simulink model "SIFT"  (R2013a)
settings: Solver=FixedStepDiscrete  SolverMode=SingleTasking  StartTime=0.0  StopTime=10.0  RelTol=1e-3
libraries: xbsIndex_r4 x365, xrbsImage_r4 x64
(part 10 of 10)

== system SIFT/Minima1/Subsystem ==
  In1 : Inport
  In2 : Inport  Port=2
  In4 : Inport  Port=3
  In6 : Inport  Port=4
  In8 : Inport  Port=5
  In10 : Inport  Port=6
  In12 : Inport  Port=7
  In14 : Inport  Port=8
  In16 : Inport  Port=9
  Relational{,1..7} (8 alike) : xbsIndex_r4/Relational  mode=a<b  en=off  latency=1  dbl_ovrd=off  block_type=relational
  Out1 : Outport
  Out2 : Outport  Port=2
  Out3 : Outport  Port=3
  Out4 : Outport  Port=4
  Out5 : Outport  Port=5
  Out6 : Outport  Port=6
  Out7 : Outport  Port=7
  Out8 : Outport  Port=8
  wires:
  In1/1 -> Relational7/1, Relational6/1, Relational5/1, Relational4/1, Relational3/1, Relational2/1, Relational1/1, Relational/1
  Relational/1 -> Out1/1
  In2/1 -> Relational/2
  In4/1 -> Relational1/2
  In6/1 -> Relational2/2
  In8/1 -> Relational3/2
  In10/1 -> Relational4/2
  In12/1 -> Relational5/2
  In14/1 -> Relational6/2
  In16/1 -> Relational7/2
  Relational2/1 -> Out3/1
  Relational1/1 -> Out2/1
  Relational3/1 -> Out4/1
  Relational4/1 -> Out5/1
  Relational6/1 -> Out7/1
  Relational5/1 -> Out6/1
  Relational7/1 -> Out8/1

== system SIFT/Minima1/Subsystem1 ==
  In1 : Inport
  In2 : Inport  Port=2
  In4 : Inport  Port=3
  In6 : Inport  Port=4
  In8 : Inport  Port=5
  In10 : Inport  Port=6
  In12 : Inport  Port=7
  In14 : Inport  Port=8
  In16 : Inport  Port=9
  Relational{,1..7} (8 alike) : xbsIndex_r4/Relational  mode=a<b  en=off  latency=1  dbl_ovrd=off  block_type=relational
  Out1 : Outport
  Out2 : Outport  Port=2
  Out3 : Outport  Port=3
  Out4 : Outport  Port=4
  Out5 : Outport  Port=5
  Out6 : Outport  Port=6
  Out7 : Outport  Port=7
  Out8 : Outport  Port=8
  wires:
  In1/1 -> Relational1/1, Relational7/1, Relational6/1, Relational5/1, Relational4/1, Relational3/1, Relational2/1, Relational/1
  Relational/1 -> Out1/1
  In2/1 -> Relational/2
  In4/1 -> Relational1/2
  In6/1 -> Relational7/2
  In8/1 -> Relational6/2
  In10/1 -> Relational5/2
  In12/1 -> Relational4/2
  In14/1 -> Relational3/2
  In16/1 -> Relational2/2
  Relational7/1 -> Out3/1
  Relational1/1 -> Out2/1
  Relational6/1 -> Out4/1
  Relational5/1 -> Out5/1
  Relational3/1 -> Out7/1
  Relational4/1 -> Out6/1
  Relational2/1 -> Out8/1

== system SIFT/Minima1/Subsystem2 ==
  In1 : Inport
  In2 : Inport  Port=2
  In4 : Inport  Port=3
  In6 : Inport  Port=4
  In8 : Inport  Port=5
  In10 : Inport  Port=6
  In12 : Inport  Port=7
  In14 : Inport  Port=8
  In16 : Inport  Port=9
  In18 : Inport  Port=10
  In20 : Inport  Port=11
  Relational{,1..9} (10 alike) : xbsIndex_r4/Relational  mode=a<b  en=off  latency=1  dbl_ovrd=off  block_type=relational
  Out1 : Outport
  Out2 : Outport  Port=2
  Out3 : Outport  Port=3
  Out4 : Outport  Port=4
  Out5 : Outport  Port=5
  Out6 : Outport  Port=6
  Out7 : Outport  Port=7
  Out8 : Outport  Port=8
  Out9 : Outport  Port=9
  Out10 : Outport  Port=10
  wires:
  In1/1 -> Relational9/1, Relational8/1, Relational7/1, Relational6/1, Relational5/1, Relational4/1, Relational3/1, Relational2/1, Relational1/1, Relational/1
  Relational/1 -> Out1/1
  In2/1 -> Relational/2
  In4/1 -> Relational1/2
  In6/1 -> Relational2/2
  In8/1 -> Relational3/2
  In10/1 -> Relational4/2
  In12/1 -> Relational5/2
  In14/1 -> Relational6/2
  In16/1 -> Relational7/2
  Relational2/1 -> Out3/1
  Relational1/1 -> Out2/1
  Relational3/1 -> Out4/1
  Relational4/1 -> Out5/1
  Relational6/1 -> Out7/1
  Relational5/1 -> Out6/1
  Relational7/1 -> Out8/1
  In18/1 -> Relational8/2
  Relational8/1 -> Out9/1
  In20/1 -> Relational9/2
  Relational9/1 -> Out10/1

== system SIFT/Gaussian Filter/Subsystem/Row1 ==
  In1 : Inport
  Demux : Demux  Outputs=5
  Out1 : Outport
  Out2 : Outport  Port=2
  Out3 : Outport  Port=3
  Out4 : Outport  Port=4
  Out5 : Outport  Port=5
  wires:
  In1/1 -> Demux/1
  Demux/1 -> Out1/1
  Demux/2 -> Out2/1
  Demux/3 -> Out3/1
  Demux/4 -> Out4/1
  Demux/5 -> Out5/1

== system SIFT/Gaussian Filter/Subsystem/Row2 ==
  In1 : Inport
  Demux : Demux  Outputs=5
  Out1 : Outport
  Out2 : Outport  Port=2
  Out3 : Outport  Port=3
  Out4 : Outport  Port=4
  Out5 : Outport  Port=5
  wires:
  In1/1 -> Demux/1
  Demux/1 -> Out1/1
  Demux/2 -> Out2/1
  Demux/3 -> Out3/1
  Demux/4 -> Out4/1
  Demux/5 -> Out5/1

== system SIFT/Gaussian Filter/Subsystem/Row3 ==
  In1 : Inport
  Demux : Demux  Outputs=5
  Out1 : Outport
  Out2 : Outport  Port=2
  Out3 : Outport  Port=3
  Out4 : Outport  Port=4
  Out5 : Outport  Port=5
  wires:
  In1/1 -> Demux/1
  Demux/1 -> Out1/1
  Demux/2 -> Out2/1
  Demux/3 -> Out3/1
  Demux/4 -> Out4/1
  Demux/5 -> Out5/1

== system SIFT/Gaussian Filter/Subsystem/Row4 ==
  In1 : Inport
  Demux : Demux  Outputs=5
  Out1 : Outport
  Out2 : Outport  Port=2
  Out3 : Outport  Port=3
  Out4 : Outport  Port=4
  Out5 : Outport  Port=5
  wires:
  In1/1 -> Demux/1
  Demux/1 -> Out1/1
  Demux/2 -> Out2/1
  Demux/3 -> Out3/1
  Demux/4 -> Out4/1
  Demux/5 -> Out5/1

== system SIFT/Gaussian Filter/Subsystem/Row5 ==
  In1 : Inport
  Demux : Demux  Outputs=5
  Out1 : Outport
  Out2 : Outport  Port=2
  Out3 : Outport  Port=3
  Out4 : Outport  Port=4
  Out5 : Outport  Port=5
  wires:
  In1/1 -> Demux/1
  Demux/1 -> Out1/1
  Demux/2 -> Out2/1
  Demux/3 -> Out3/1
  Demux/4 -> Out4/1
  Demux/5 -> Out5/1

== system SIFT/Gaussian Filter1/Subsystem/Row1 ==
  In1 : Inport
  Demux : Demux  Outputs=5
  Out1 : Outport
  Out2 : Outport  Port=2
  Out3 : Outport  Port=3
  Out4 : Outport  Port=4
  Out5 : Outport  Port=5
  wires:
  In1/1 -> Demux/1
  Demux/1 -> Out1/1
  Demux/2 -> Out2/1
  Demux/3 -> Out3/1
  Demux/4 -> Out4/1
  Demux/5 -> Out5/1

== system SIFT/Gaussian Filter1/Subsystem/Row2 ==
  In1 : Inport
  Demux : Demux  Outputs=5
  Out1 : Outport
  Out2 : Outport  Port=2
  Out3 : Outport  Port=3
  Out4 : Outport  Port=4
  Out5 : Outport  Port=5
  wires:
  In1/1 -> Demux/1
  Demux/1 -> Out1/1
  Demux/2 -> Out2/1
  Demux/3 -> Out3/1
  Demux/4 -> Out4/1
  Demux/5 -> Out5/1

== system SIFT/Gaussian Filter1/Subsystem/Row3 ==
  In1 : Inport
  Demux : Demux  Outputs=5
  Out1 : Outport
  Out2 : Outport  Port=2
  Out3 : Outport  Port=3
  Out4 : Outport  Port=4
  Out5 : Outport  Port=5
  wires:
  In1/1 -> Demux/1
  Demux/1 -> Out1/1
  Demux/2 -> Out2/1
  Demux/3 -> Out3/1
  Demux/4 -> Out4/1
  Demux/5 -> Out5/1

== system SIFT/Gaussian Filter1/Subsystem/Row4 ==
  In1 : Inport
  Demux : Demux  Outputs=5
  Out1 : Outport
  Out2 : Outport  Port=2
  Out3 : Outport  Port=3
  Out4 : Outport  Port=4
  Out5 : Outport  Port=5
  wires:
  In1/1 -> Demux/1
  Demux/1 -> Out1/1
  Demux/2 -> Out2/1
  Demux/3 -> Out3/1
  Demux/4 -> Out4/1
  Demux/5 -> Out5/1

== system SIFT/Gaussian Filter1/Subsystem/Row5 ==
  In1 : Inport
  Demux : Demux  Outputs=5
  Out1 : Outport
  Out2 : Outport  Port=2
  Out3 : Outport  Port=3
  Out4 : Outport  Port=4
  Out5 : Outport  Port=5
  wires:
  In1/1 -> Demux/1
  Demux/1 -> Out1/1
  Demux/2 -> Out2/1
  Demux/3 -> Out3/1
  Demux/4 -> Out4/1
  Demux/5 -> Out5/1

== system SIFT/Gaussian Filter2/Subsystem/Row1 ==
  In1 : Inport
  Demux : Demux  Outputs=5
  Out1 : Outport
  Out2 : Outport  Port=2
  Out3 : Outport  Port=3
  Out4 : Outport  Port=4
  Out5 : Outport  Port=5
  wires:
  In1/1 -> Demux/1
  Demux/1 -> Out1/1
  Demux/2 -> Out2/1
  Demux/3 -> Out3/1
  Demux/4 -> Out4/1
  Demux/5 -> Out5/1

== system SIFT/Gaussian Filter2/Subsystem/Row2 ==
  In1 : Inport
  Demux : Demux  Outputs=5
  Out1 : Outport
  Out2 : Outport  Port=2
  Out3 : Outport  Port=3
  Out4 : Outport  Port=4
  Out5 : Outport  Port=5
  wires:
  In1/1 -> Demux/1
  Demux/1 -> Out1/1
  Demux/2 -> Out2/1
  Demux/3 -> Out3/1
  Demux/4 -> Out4/1
  Demux/5 -> Out5/1

== system SIFT/Gaussian Filter2/Subsystem/Row3 ==
  In1 : Inport
  Demux : Demux  Outputs=5
  Out1 : Outport
  Out2 : Outport  Port=2
  Out3 : Outport  Port=3
  Out4 : Outport  Port=4
  Out5 : Outport  Port=5
  wires:
  In1/1 -> Demux/1
  Demux/1 -> Out1/1
  Demux/2 -> Out2/1
  Demux/3 -> Out3/1
  Demux/4 -> Out4/1
  Demux/5 -> Out5/1

== system SIFT/Gaussian Filter2/Subsystem/Row4 ==
  In1 : Inport
  Demux : Demux  Outputs=5
  Out1 : Outport
  Out2 : Outport  Port=2
  Out3 : Outport  Port=3
  Out4 : Outport  Port=4
  Out5 : Outport  Port=5
  wires:
  In1/1 -> Demux/1
  Demux/1 -> Out1/1
  Demux/2 -> Out2/1
  Demux/3 -> Out3/1
  Demux/4 -> Out4/1
  Demux/5 -> Out5/1

== system SIFT/Gaussian Filter2/Subsystem/Row5 ==
  In1 : Inport
  Demux : Demux  Outputs=5
  Out1 : Outport
  Out2 : Outport  Port=2
  Out3 : Outport  Port=3
  Out4 : Outport  Port=4
  Out5 : Outport  Port=5
  wires:
  In1/1 -> Demux/1
  Demux/1 -> Out1/1
  Demux/2 -> Out2/1
  Demux/3 -> Out3/1
  Demux/4 -> Out4/1
  Demux/5 -> Out5/1

== system SIFT/Gaussian Filter3/Subsystem/Row1 ==
  In1 : Inport
  Demux : Demux  Outputs=5
  Out1 : Outport
  Out2 : Outport  Port=2
  Out3 : Outport  Port=3
  Out4 : Outport  Port=4
  Out5 : Outport  Port=5
  wires:
  In1/1 -> Demux/1
  Demux/1 -> Out1/1
  Demux/2 -> Out2/1
  Demux/3 -> Out3/1
  Demux/4 -> Out4/1
  Demux/5 -> Out5/1

== system SIFT/Gaussian Filter3/Subsystem/Row2 ==
  In1 : Inport
  Demux : Demux  Outputs=5
  Out1 : Outport
  Out2 : Outport  Port=2
  Out3 : Outport  Port=3
  Out4 : Outport  Port=4
  Out5 : Outport  Port=5
  wires:
  In1/1 -> Demux/1
  Demux/1 -> Out1/1
  Demux/2 -> Out2/1
  Demux/3 -> Out3/1
  Demux/4 -> Out4/1
  Demux/5 -> Out5/1

== system SIFT/Gaussian Filter3/Subsystem/Row3 ==
  In1 : Inport
  Demux : Demux  Outputs=5
  Out1 : Outport
  Out2 : Outport  Port=2
  Out3 : Outport  Port=3
  Out4 : Outport  Port=4
  Out5 : Outport  Port=5
  wires:
  In1/1 -> Demux/1
  Demux/1 -> Out1/1
  Demux/2 -> Out2/1
  Demux/3 -> Out3/1
  Demux/4 -> Out4/1
  Demux/5 -> Out5/1

== system SIFT/Gaussian Filter3/Subsystem/Row4 ==
  In1 : Inport
  Demux : Demux  Outputs=5
  Out1 : Outport
  Out2 : Outport  Port=2
  Out3 : Outport  Port=3
  Out4 : Outport  Port=4
  Out5 : Outport  Port=5
  wires:
  In1/1 -> Demux/1
  Demux/1 -> Out1/1
  Demux/2 -> Out2/1
  Demux/3 -> Out3/1
  Demux/4 -> Out4/1
  Demux/5 -> Out5/1

== system SIFT/Gaussian Filter3/Subsystem/Row5 ==
  In1 : Inport
  Demux : Demux  Outputs=5
  Out1 : Outport
  Out2 : Outport  Port=2
  Out3 : Outport  Port=3
  Out4 : Outport  Port=4
  Out5 : Outport  Port=5
  wires:
  In1/1 -> Demux/1
  Demux/1 -> Out1/1
  Demux/2 -> Out2/1
  Demux/3 -> Out3/1
  Demux/4 -> Out4/1
  Demux/5 -> Out5/1

== system SIFT/Gaussian Filter4/Subsystem/Row1 ==
  In1 : Inport
  Demux : Demux  Outputs=5
  Out1 : Outport
  Out2 : Outport  Port=2
  Out3 : Outport  Port=3
  Out4 : Outport  Port=4
  Out5 : Outport  Port=5
  wires:
  In1/1 -> Demux/1
  Demux/1 -> Out1/1
  Demux/2 -> Out2/1
  Demux/3 -> Out3/1
  Demux/4 -> Out4/1
  Demux/5 -> Out5/1

== system SIFT/Gaussian Filter4/Subsystem/Row2 ==
  In1 : Inport
  Demux : Demux  Outputs=5
  Out1 : Outport
  Out2 : Outport  Port=2
  Out3 : Outport  Port=3
  Out4 : Outport  Port=4
  Out5 : Outport  Port=5
  wires:
  In1/1 -> Demux/1
  Demux/1 -> Out1/1
  Demux/2 -> Out2/1
  Demux/3 -> Out3/1
  Demux/4 -> Out4/1
  Demux/5 -> Out5/1

== system SIFT/Gaussian Filter4/Subsystem/Row3 ==
  In1 : Inport
  Demux : Demux  Outputs=5
  Out1 : Outport
  Out2 : Outport  Port=2
  Out3 : Outport  Port=3
  Out4 : Outport  Port=4
  Out5 : Outport  Port=5
  wires:
  In1/1 -> Demux/1
  Demux/1 -> Out1/1
  Demux/2 -> Out2/1
  Demux/3 -> Out3/1
  Demux/4 -> Out4/1
  Demux/5 -> Out5/1

== system SIFT/Gaussian Filter4/Subsystem/Row4 ==
  In1 : Inport
  Demux : Demux  Outputs=5
  Out1 : Outport
  Out2 : Outport  Port=2
  Out3 : Outport  Port=3
  Out4 : Outport  Port=4
  Out5 : Outport  Port=5
  wires:
  In1/1 -> Demux/1
  Demux/1 -> Out1/1
  Demux/2 -> Out2/1
  Demux/3 -> Out3/1
  Demux/4 -> Out4/1
  Demux/5 -> Out5/1

== system SIFT/Gaussian Filter4/Subsystem/Row5 ==
  In1 : Inport
  Demux : Demux  Outputs=5
  Out1 : Outport
  Out2 : Outport  Port=2
  Out3 : Outport  Port=3
  Out4 : Outport  Port=4
  Out5 : Outport  Port=5
  wires:
  In1/1 -> Demux/1
  Demux/1 -> Out1/1
  Demux/2 -> Out2/1
  Demux/3 -> Out3/1
  Demux/4 -> Out4/1
  Demux/5 -> Out5/1

== system SIFT/Gaussian Filter5/Subsystem/Row1 ==
  In1 : Inport
  Demux : Demux  Outputs=5
  Out1 : Outport
  Out2 : Outport  Port=2
  Out3 : Outport  Port=3
  Out4 : Outport  Port=4
  Out5 : Outport  Port=5
  wires:
  In1/1 -> Demux/1
  Demux/1 -> Out1/1
  Demux/2 -> Out2/1
  Demux/3 -> Out3/1
  Demux/4 -> Out4/1
  Demux/5 -> Out5/1

== system SIFT/Gaussian Filter5/Subsystem/Row2 ==
  In1 : Inport
  Demux : Demux  Outputs=5
  Out1 : Outport
  Out2 : Outport  Port=2
  Out3 : Outport  Port=3
  Out4 : Outport  Port=4
  Out5 : Outport  Port=5
  wires:
  In1/1 -> Demux/1
  Demux/1 -> Out1/1
  Demux/2 -> Out2/1
  Demux/3 -> Out3/1
  Demux/4 -> Out4/1
  Demux/5 -> Out5/1

== system SIFT/Gaussian Filter5/Subsystem/Row3 ==
  In1 : Inport
  Demux : Demux  Outputs=5
  Out1 : Outport
  Out2 : Outport  Port=2
  Out3 : Outport  Port=3
  Out4 : Outport  Port=4
  Out5 : Outport  Port=5
  wires:
  In1/1 -> Demux/1
  Demux/1 -> Out1/1
  Demux/2 -> Out2/1
  Demux/3 -> Out3/1
  Demux/4 -> Out4/1
  Demux/5 -> Out5/1

== system SIFT/Gaussian Filter5/Subsystem/Row4 ==
  In1 : Inport
  Demux : Demux  Outputs=5
  Out1 : Outport
  Out2 : Outport  Port=2
  Out3 : Outport  Port=3
  Out4 : Outport  Port=4
  Out5 : Outport  Port=5
  wires:
  In1/1 -> Demux/1
  Demux/1 -> Out1/1
  Demux/2 -> Out2/1
  Demux/3 -> Out3/1
  Demux/4 -> Out4/1
  Demux/5 -> Out5/1

== system SIFT/Gaussian Filter5/Subsystem/Row5 ==
  In1 : Inport
  Demux : Demux  Outputs=5
  Out1 : Outport
  Out2 : Outport  Port=2
  Out3 : Outport  Port=3
  Out4 : Outport  Port=4
  Out5 : Outport  Port=5
  wires:
  In1/1 -> Demux/1
  Demux/1 -> Out1/1
  Demux/2 -> Out2/1
  Demux/3 -> Out3/1
  Demux/4 -> Out4/1
  Demux/5 -> Out5/1
